simulink model "satellite_formation_control"  (R2022b)
settings: Solver=VariableStepAuto  StartTime=0.0  StopTime=500  RelTol=1e-3
values from neighbouring files (symbols this model uses):
  Km = kron(L,-c*B*K)    [stable_consensus.m]
  x0 = [x1_0 ... (first row only)    [stable_consensus.m]
  x1_0 = [0 500 866*sqrt(3) 1.5 0 0].'    [stable_consensus.m]
  xd = [x1d, x2d, x3d, x4d, x5d, x6d]    [Plot_results.m]    (also in stable_consensus.m = [x1d)
settings Model: Creator=yu zheng  LastModifiedBy=Abelb
settings SolverCC: AlgebraicLoopSolver=TrustRegion
settings DebuggingCC: UnconnectedInputMsg=warning  UnconnectedOutputMsg=warning  UnconnectedLineMsg=warning  SFMachineParentedDataDiag=warning
settings ModelReferenceCC: EnableRefExpFcnMdlSchedulingChecks=on
settings RTWCC: DLArmComputeVersion=19.05

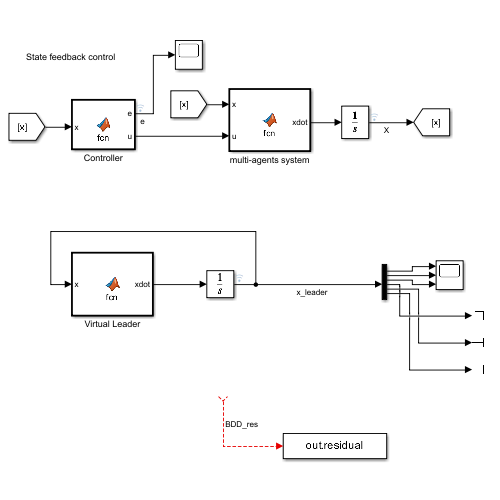
[thumbnail: Simulink's stored preview of the top-level diagram]
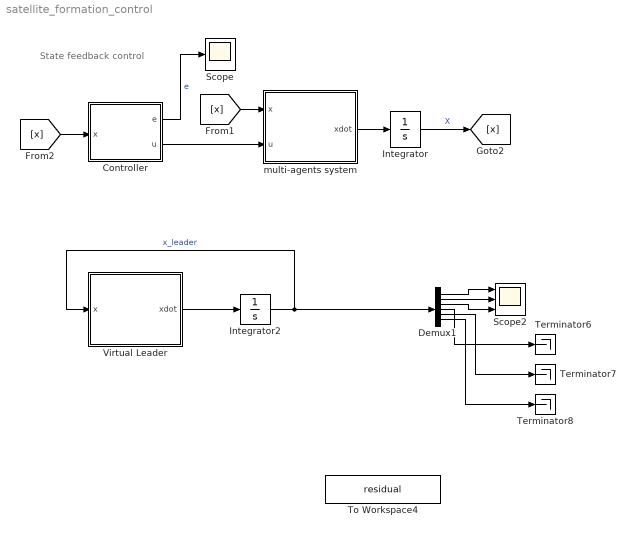
== system satellite_formation_control ==
  note: State feedback control
  Controller : MATLAB Function  TreatAsAtomicUnit=on
  Demux1 : Demux  Outputs=6
  Integrator : Integrator  InitialCondition=x0
  Integrator2 : Integrator  InitialCondition=x1_0
  Scope : Scope
  Scope2 : Scope  NumInputPorts=3
  Terminator6 : Terminator
  Terminator7 : Terminator
  Terminator8 : Terminator
  To Workspace4 : ToWorkspace  VariableName=residual  SaveFormat=Timeseries  SampleTime=-1
  Virtual Leader : MATLAB Function  TreatAsAtomicUnit=on
  multi-agents system : MATLAB Function  TreatAsAtomicUnit=on
  wires:
  multi-agents system/1(xdot) -> Integrator/1
  Integrator/1 -> [x]  "X"
  Controller/2(u) -> multi-agents system/2(u)
  Virtual Leader/1(xdot) -> Integrator2/1
  Demux1/4 -> Terminator6/1
  Demux1/1 -> Scope2/1
  Demux1/2 -> Scope2/2
  Integrator2/1 -> Virtual Leader/1(x), Demux1/1  "x_leader"
  Demux1/3 -> Scope2/3
  Demux1/6 -> Terminator8/1
  Demux1/5 -> Terminator7/1
  [x] -> multi-agents system/1(x)
  [x] -> Controller/1(x)
  Controller/1(e) -> Scope/1  "e"
  ? -> To Workspace4/1  "BDD_res"

== matlab function satellite_formation_control/Controller ==
  data: e output; x input; u output; xd parameter; Km parameter
function [e,u] = fcn(x,xd,Km)

% x1 = x(1:n);
% x2 = x(n+1:2*n);
% x3 = x(2*n+1:3*n);
% x4 = x(3*n+1:4*n);
% x5 = x(4*n+1:5*n);
% x6 = x(5*n+1:6*n);

% e = Um*(x-xd);
e = x-xd;
u = Km*(x-xd);
u(1:6)=zeros(6,1);

== matlab function satellite_formation_control/multi-agents system ==
  data: x input; u input; xdot output; Am parameter
function xdot = fcn(x,u,Am)


xdot = Am*x +u ;

== matlab function satellite_formation_control/Virtual Leader ==
  data: x input; xdot output; A parameter
function xdot = fcn(x, A)

n = size(A,1);
xdot = A*x ;
